simulink model "Object-Detection"  (R2021b)
settings: Solver=FixedStepAuto  StartTime=0.0  StopTime=20.0  RelTol=1e-3  EnableMultiTasking=on
libraries: legoev3lib x4, simulink x2, simulink_extras x2
settings Model: ExtModeTrigDuration=2  Creator=s142  LastModifiedBy=s142
settings SolverCC: PositivePriorityOrder=on
settings OptimizationCC: EnhancedBackFolding=on  PassReuseOutputArgsAs=Individual arguments  ZeroExternalMemoryAtStartup=off  ZeroInternalMemoryAtStartup=off  MaxStackSize=64  OptimizeBlockOrder=speed  DifferentSizesBufferReuse=on  OptimizationCustomize=off  EfficientTunableParamExpr=on
settings DebuggingCC: ParameterTunabilityLossMsg=error
settings HardwareCC: ProdBitPerPointer=32  ProdBitPerSizeT=32  ProdBitPerPtrDiffT=32  ProdLargestAtomicInteger=Long  ProdWordSize=32  ProdHWDeviceType=ARM Compatible->ARM 9
settings SFSimCC: MATLABDynamicMemAlloc=off
settings RTWCC: Description=Embedded Coder  SystemTargetFile=ert.tlc  HardwareBoard=LEGO MINDSTORMS EV3  TLCOptions="-aInlineSetEventsForThisBaseRateFcn=TLC_FALSE -aSuppressMultiTaskScheduler=TLC_FALSE  -aRateBasedStepFcn=0"  TemplateMakefile=ert_default_tmf  Toolchain=Sourcery G++ Lite v2009q3
settings CodeAppCC: ForceParamTrailComments=on  IgnoreCustomStorageClasses=off  OperatorAnnotations=on  SimulinkDataObjDesc=on  SFDataObjDesc=on  InsertBlockDesc=on
settings ERTTargetCC: SupportContinuousTime=on  SupportVariableSizeSignals=on  ExtModeTransport=2  ExtModeStaticAlloc=on  ExtModeMexFile=ext_xcp  ExtModeIntrfLevel=Level2 - Open

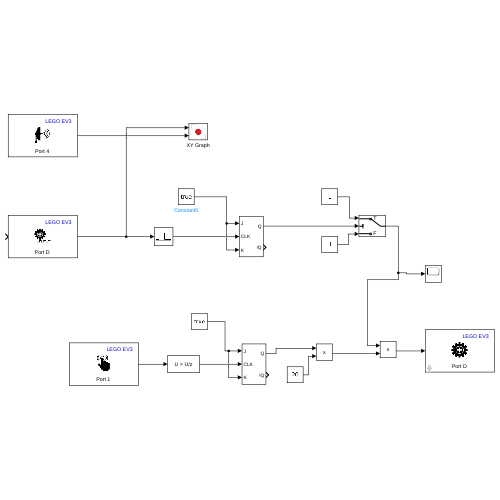
[thumbnail: Simulink's stored preview of the top-level diagram]
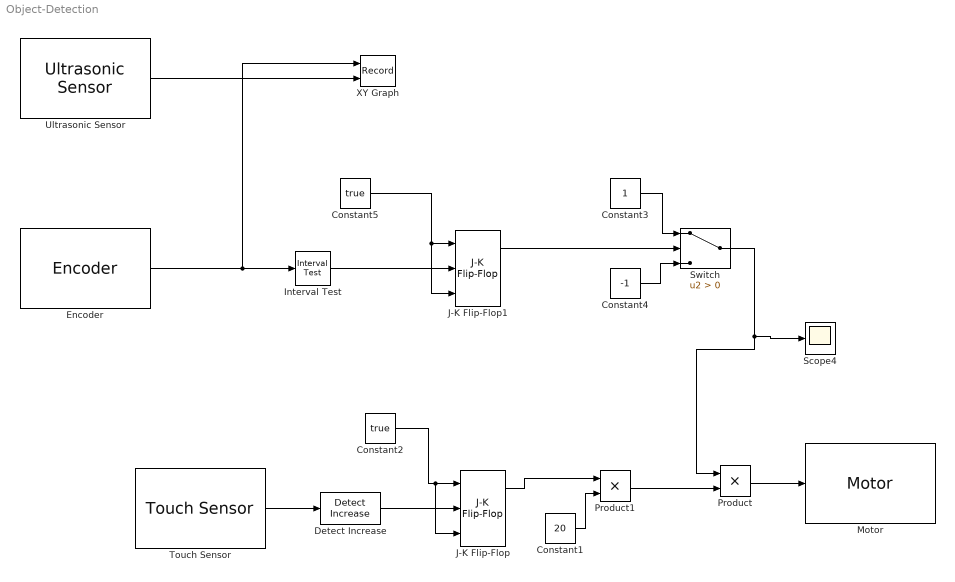
== system Object-Detection ==
  Constant1 : Constant  Value=20
  Constant2 : Constant  Value=true  OutDataTypeStr=boolean
  Constant3 : Constant
  Constant4 : Constant  Value=-1
  Constant5 : Constant  Value=true  OutDataTypeStr=boolean
  Detect Increase : simulink/Logic and Bit Operations/Detect Increase  vinit=0.0  OutDataTypeStr=boolean
  Encoder : legoev3lib/Encoder  portNumber=D  opMode=Reset by external signal  sampleTime=0.01
      settings: SourceProductBaseCode=LEGOEV3
  Interval Test : simulink/Logic and Bit Operations/Interval Test  IntervalClosedRight=on  uplimit=60  IntervalClosedLeft=on  lowlimit=-60  OutDataTypeStr=boolean
  J-K Flip-Flop : simulink_extras/Flip Flops/J-K Flip-Flop  initial_condition=0
  J-K Flip-Flop1 : simulink_extras/Flip Flops/J-K Flip-Flop  initial_condition=0
  Motor : legoev3lib/Motor  sportNumber=D  sstopAction=Brake
  Product : Product
  Product1 : Product
  Scope4 : Scope
  Switch : Switch  Criteria=u2 > Threshold
  Touch Sensor : legoev3lib/Touch Sensor  portNumber=1  sampleTime=0.01
      settings: SourceProductBaseCode=LEGOEV3
  Ultrasonic Sensor : legoev3lib/Ultrasonic Sensor  PortNumber=4  sampleTime=0.01
      settings: SourceProductBaseCode=LEGOEV3
  XY Graph : Record  FileSettingsInternal="{\"entries\":[{\"content\":{\"excelSettings\":{\"content\":{},\"type\":\"Streamout.ExcelSettings\"}},\"type\":\"Streamout.FileSettingStorage\",\"uuid\":\"0d61d9b8-e41d-4b6d-b978-dd19d6224bbf\"}],\"packageUris\":[\"http://schema.mathworks.com/mf0/streamout_blocks/R2020a\"],\"version\":\"1.0\"}"  Layout=[1 1]  SignalsInternal="{\"entries\":[{\"content\":{\"signals\":[{\"content\":{\"blockPath\":[\"exercise_32/XY Graph\"],\"channel\":[],\"dimensions\":[1],\"domain\":\"exercise_32/XY Graph\",\"lineColor\":\"#139fff\",\"plots\":[1],\"port\":2,\"sid\":[\"19\"],\"signalID\":55031,\"signalName\":\"Ultrasonic Sensor\"},\"type\":\"RecordBlkView.Signal\",\"uuid\":\"5f5e26c7-c931-410d-8c5a-c5322973e894\"},{\"content\":{\"blockPath\":[\"exercise_32/XY Graph\"],\"channel\":[],\"dimensions\":[1],\"domain\":\"exercise_32/XY Graph\",\"lineColor\":\"#a2142f\",\"plots\":[1],\"port\":1,\"sid\":[\"19\"],\"signalID\":55039,\"signalName\":\"Encoder\"},\"type\":\"RecordBlkView.Signal\",\"uuid\":\"a9fef2b7-8702-46e9-9907-10274498f747\"}]},\"type\":\"RecordBlkView.InputSignals\",\"uuid\":\"fdfceab1-a11b-4c3f-9601-ea0a5759a961\"}],\"packageUris\":[\"http://schema.mathworks.com/mf0/streamout_blocks/R2020a\"],\"version\":\"1.0\"}"  VisualizationBindings="{\"xyplotplugin\":{\"info\":[{\"series\":[{\"bindingParametersList\":[{\"parameter\":\"X-Axis\",\"signalID\":55039,\"signalName\":\"Encoder\"},{\"parameter\":\"Y-Axis\",\"signalID\":55031,\"signalName\":\"Ultrasonic Sensor\"}],\"seriesID\":52265}],\"subplotID\":1}]}}"  CompatibilityTag=XY
  wires:
  Detect Increase/1 -> J-K Flip-Flop/2
  Switch/1 -> Scope4/1, Product/1
  J-K Flip-Flop1/1 -> Switch/2
  Touch Sensor/1 -> Detect Increase/1
  Interval Test/1 -> J-K Flip-Flop1/2
  J-K Flip-Flop/1 -> Product1/1
  Encoder/1 -> XY Graph/1, Interval Test/1
  Product/1 -> Motor/1
  Constant4/1 -> Switch/3
  Constant3/1 -> Switch/1
  Product1/1 -> Product/2
  Constant1/1 -> Product1/2
  Constant2/1 -> J-K Flip-Flop/3, J-K Flip-Flop/1
  Constant5/1 -> J-K Flip-Flop1/3, J-K Flip-Flop1/1
  Ultrasonic Sensor/1 -> XY Graph/2
